simulink model "Improved_EKFSim"  (R2023b)
settings: Solver=VariableStepAuto  StartTime=0.0  StopTime=6000  RelTol=1e-3
libraries: commchan3 x2, SignalEditorBlockLib x1
settings Model: Creator=Lenovo  LastModifiedBy=dell
settings SolverCC: AlgebraicLoopSolver=TrustRegion
settings DataIOCC: ReturnWorkspaceOutputs=off
settings DebuggingCC: UnconnectedInputMsg=warning  UnconnectedOutputMsg=warning  UnconnectedLineMsg=warning  ArithmeticOperatorsInVariantConditions=warning
settings ModelReferenceCC: EnableRefExpFcnMdlSchedulingChecks=on
settings SFSimCC: SimUseLocalCustomCode=off  CustomCodeUndefinedFunction=UseInterfaceOnly
settings RTWCC: RTWUseLocalCustomCode=off  DLArmComputeVersion=19.05

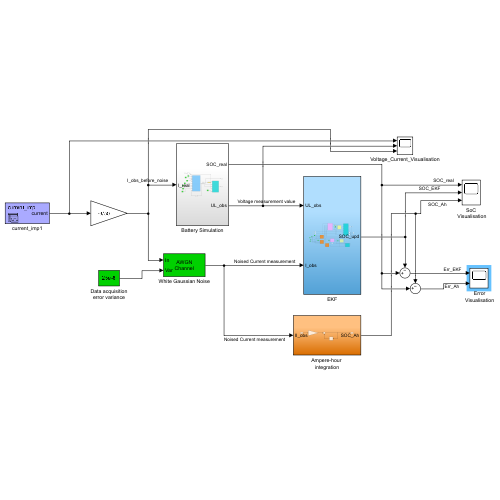
[thumbnail: Simulink's stored preview of the top-level diagram]
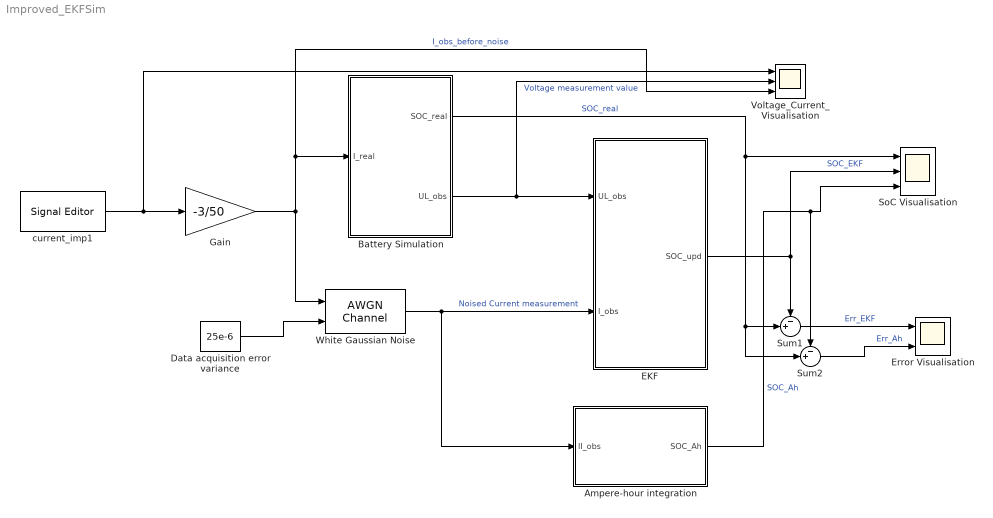
== system Improved_EKFSim ==
  "  Error Visualisation" : Scope  NumInputPorts=2
  " SoC Visualisation" : Scope  NumInputPorts=3
  Ampere-hour integration : Subsystem
  Battery Simulation : Subsystem
  Data acquisition error variance : Constant  Value=25e-6
  EKF : Subsystem
  Gain : Gain  Gain=-3/50
  Sum1 : Sum  Inputs=-+|
  Sum2 : Sum  Inputs=-+|
  Voltage_Current_Visualisation : Scope  NumInputPorts=3
  White Gaussian Noise : commchan3/AWGN Channel  LegacyMode=on  NoiseMethod="Signal to noise ratio  (SNR)"  noiseMode=Variance from port  EbNo=10  EsNo=10  SNR=10  BitsPerSymbol=1  SignalPower=1  SamplesPerSymbol=1  SymbolPeriod=1  VarianceSource=Parameter  Variance=1  RandomStream=Global stream  Seed=1  SimulateUsing=Code generation
  current_imp1 : SignalEditorBlockLib/Signal Editor  FileName=C:\Users\dell\Downloads\BMS_EKF\scripts\dataset.mat  ActiveScenario=current_imp  ActiveSignal=current  IsBus=off  OutputBusObjectStr=Bus: BusObject  SampleTime=0  OutputAfterFinalValue=Extrapolation  Unit=inherit  PreserveSignalName=on  ApplySigPropsToAllScenarios=on  ApplySigPropsToAllSignals=off
  wires:
  White Gaussian Noise/1 -> EKF/2(I_obs), Ampere-hour integration/1(II_obs)  "Noised Current measurement"
  EKF/1(SOC_upd) -> Sum1/1, " SoC Visualisation"/2  "SOC_EKF"
  Battery Simulation/2(UL_obs) -> Voltage_Current_Visualisation/2, EKF/1(UL_obs)  "Voltage measurement value"
  Battery Simulation/1(SOC_real) -> Sum2/2, Sum1/2, " SoC Visualisation"/1  "SOC_real"
  Gain/1 -> Voltage_Current_Visualisation/3, Battery Simulation/1(I_real), White Gaussian Noise/1  "I_obs_before_noise"
  Ampere-hour integration/1(SOC_Ah) -> " SoC Visualisation"/3, Sum2/1  "SOC_Ah"
  Sum1/1 -> "  Error Visualisation"/1  "Err_EKF"
  Sum2/1 -> "  Error Visualisation"/2  "Err_Ah"
  Data acquisition error variance/1 -> White Gaussian Noise/2
  current_imp1/1 -> Voltage_Current_Visualisation/1, Gain/1

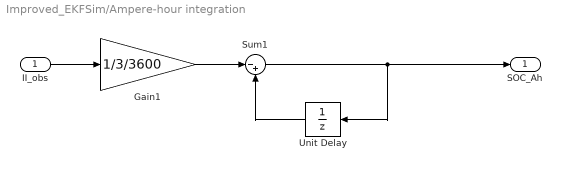
== system Improved_EKFSim/Ampere-hour integration ==
  II_obs : Inport
  Gain1 : Gain  Gain=1/3/3600
  Sum1 : Sum  Inputs=|-+
  Unit Delay : UnitDelay  InitialCondition=1  HasFrameUpgradeWarning=on
  SOC_Ah : Outport  VectorParamsAs1DForOutWhenUnconnected=off
  wires:
  Gain1/1 -> Sum1/1
  Sum1/1 -> SOC_Ah/1, Unit Delay/1
  II_obs/1 -> Gain1/1
  Unit Delay/1 -> Sum1/2

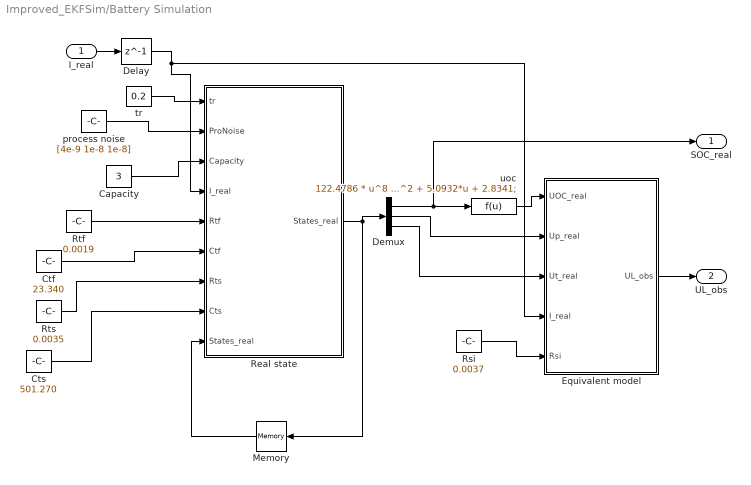
== system Improved_EKFSim/Battery Simulation ==
  I_real : Inport
  Capacity : Constant  Value=3
  Ctf : Constant  Value=23.340
  Cts : Constant  Value=501.270
  Delay : Delay  DelayLength=1  InitialCondition=0  SampleTime=0.1
  Demux : Demux  Outputs=3
  Equivalent model : Subsystem  TreatAsAtomicUnit=on
  Memory : Memory  InitialCondition=[1;0;0]
  Real state : MATLAB Function  TreatAsAtomicUnit=on
  Rsi : Constant  Value=0.0037
  Rtf : Constant  Value=0.0019
  Rts : Constant  Value=0.0035
  process noise : Constant  Value=[4e-9 1e-8 1e-8]
  tr : Constant  Value=0.2
  uoc : Fcn  Expr=122.4786 * u^8 - 401.4734 * u^7 + 485.6818 * u^6 -239.2806 * u^5 + 3.7304 * u^4 + 44.9020 * u^3 - 19.8057 * u^2 + 5.0932*u + 2.8341;
  SOC_real : Outport  VectorParamsAs1DForOutWhenUnconnected=off
  UL_obs : Outport  Port=2  VectorParamsAs1DForOutWhenUnconnected=off
  wires:
  Demux/2 -> Equivalent model/2(Up_real)
  Rtf/1 -> Real state/5(Rtf)
  tr/1 -> Real state/1(tr)
  Real state/1(States_real) -> Demux/1, Memory/1
  Rsi/1 -> Equivalent model/5(Rsi)
  Ctf/1 -> Real state/6(Ctf)
  Capacity/1 -> Real state/3(Capacity)
  uoc/1 -> Equivalent model/1(UOC_real)
  Memory/1 -> Real state/9("States_real ")
  process noise/1 -> Real state/2(ProNoise)
  Equivalent model/1(UL_obs) -> UL_obs/1
  Delay/1 -> Real state/4(I_real), Equivalent model/4(I_real)
  Demux/1 -> uoc/1, SOC_real/1
  I_real/1 -> Delay/1
  Rts/1 -> Real state/7(Rts)
  Cts/1 -> Real state/8(Cts)
  Demux/3 -> Equivalent model/3(Ut_real)

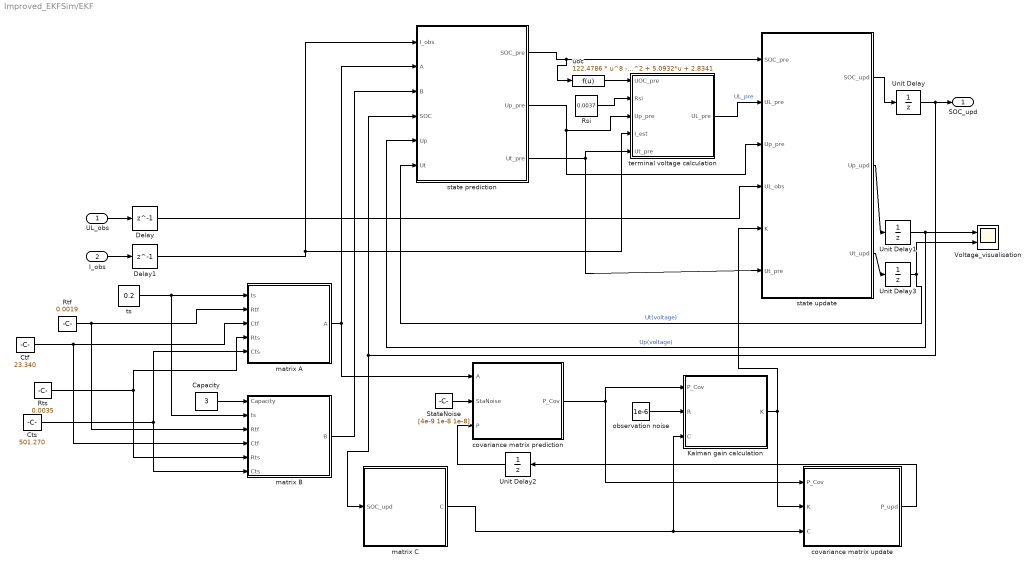
== system Improved_EKFSim/EKF ==
  UL_obs : Inport
  I_obs : Inport  Port=2
  Capacity : Constant  Value=3
  Ctf : Constant  Value=23.340
  Cts : Constant  Value=501.270
  Delay : Delay  DelayLength=1  InitialCondition=0  SampleTime=1
  Delay1 : Delay  DelayLength=1  InitialCondition=0  SampleTime=1
  Kalman gain calculation : MATLAB Function  TreatAsAtomicUnit=on
  Rsi : Constant  Value=0.0037
  Rtf : Constant  Value=0.0019
  Rts : Constant  Value=0.0035
  StateNoise : Constant  Value=[4e-9 1e-8 1e-8]
  Unit Delay : UnitDelay  InitialCondition=1  HasFrameUpgradeWarning=on
  Unit Delay1 : UnitDelay  HasFrameUpgradeWarning=on
  Unit Delay2 : UnitDelay  InitialCondition=[0 0 0;0 0 0; 0 0 0]  HasFrameUpgradeWarning=on
  Unit Delay3 : UnitDelay  HasFrameUpgradeWarning=on
  Voltage_visualisation : Scope  NumInputPorts=2
  covariance matrix prediction : MATLAB Function  TreatAsAtomicUnit=on
  covariance matrix update : MATLAB Function  TreatAsAtomicUnit=on
  matrix A : Subsystem  TreatAsAtomicUnit=on
  matrix B : Subsystem  TreatAsAtomicUnit=on
  matrix C : Subsystem  TreatAsAtomicUnit=on
  observation noise : Constant  Value=1e-6
  state prediction : Subsystem
  state update : Subsystem
  terminal voltage calculation : Subsystem  TreatAsAtomicUnit=on
  ts : Constant  Value=0.2
  uoc : Fcn  Expr=122.4786 * u^8 - 401.4734 * u^7 + 485.6818 * u^6 -239.2806 * u^5 + 3.7304 * u^4 + 44.9020 * u^3 - 19.8057 * u^2 + 5.0932*u + 2.8341
  SOC_upd : Outport  VectorParamsAs1DForOutWhenUnconnected=off
  wires:
  matrix C/1(" C") -> covariance matrix update/3(C), Kalman gain calculation/3(C)
  matrix A/1(A) -> state prediction/2(A), covariance matrix prediction/1(A)
  StateNoise/1 -> covariance matrix prediction/2(StaNoise)
  Kalman gain calculation/1(K) -> covariance matrix update/2(K), state update/5(K)
  ts/1 -> matrix B/2(ts), matrix A/1(ts)
  covariance matrix update/1(P_upd) -> Unit Delay2/1
  Capacity/1 -> matrix B/1(Capacity)
  I_obs/1 -> Delay1/1
  observation noise/1 -> Kalman gain calculation/2(R)
  UL_obs/1 -> Delay/1
  uoc/1 -> terminal voltage calculation/1(UOC_pre)
  Delay1/1 -> state prediction/1(I_obs), terminal voltage calculation/4(I_est)
  state update/2(Up_upd) -> Unit Delay1/1
  state update/1(SOC_upd) -> Unit Delay/1
  terminal voltage calculation/1(UL_pre) -> state update/2(UL_pre)  "UL_pre"
  Delay/1 -> state update/4(UL_obs)
  state prediction/1(SOC_pre) -> uoc/1, state update/1(SOC_pre)
  state prediction/2(Up_pre) -> state update/3(Up_pre), terminal voltage calculation/3(Up_pre)
  Unit Delay/1 -> state prediction/4(SOC), matrix C/1(SOC_upd), SOC_upd/1
  Unit Delay1/1 -> state prediction/5(Up), Voltage_visualisation/1  "Up(voltage)"
  matrix B/1(B) -> state prediction/3(B)
  covariance matrix prediction/1(P_Cov) -> covariance matrix update/1(P_Cov), Kalman gain calculation/1(P_Cov)
  Unit Delay2/1 -> covariance matrix prediction/3(P)
  Rtf/1 -> matrix B/3(Rtf), matrix A/2(Rtf)
  Ctf/1 -> matrix B/4(Ctf), matrix A/3(Ctf)
  Rts/1 -> matrix A/4(Rts), matrix B/5(Rts)
  Cts/1 -> matrix B/6(Cts), matrix A/5(Cts)
  Rsi/1 -> terminal voltage calculation/2(Rsi)
  state prediction/3(Ut_pre) -> state update/6(Ut_pre), terminal voltage calculation/5(Ut_pre)
  state update/3(Ut_upd) -> Unit Delay3/1
  Unit Delay3/1 -> Voltage_visualisation/2, state prediction/6(Ut)  "Ut(voltage)"

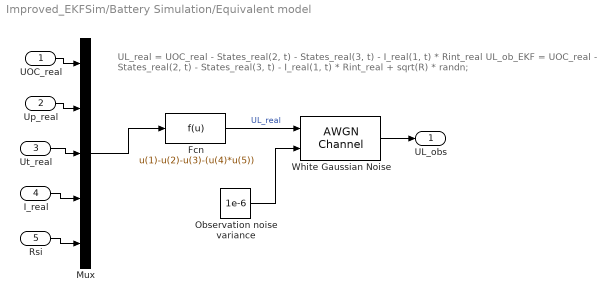
== system Improved_EKFSim/Battery Simulation/Equivalent model ==
  note: UL_real = UOC_real - States_real(2, t) - States_real(3, t) - I_real(1, t) * Rint_real
      | UL_ob_EKF = UOC_real - States_real(2, t) - States_real(3, t) - I_real(1, t) * Rint_real + sqrt(R) * randn;
  UOC_real : Inport
  Up_real : Inport  Port=2
  Ut_real : Inport  Port=3
  I_real : Inport  Port=4
  Rsi : Inport  Port=5
  Fcn : Fcn  Expr=u(1)-u(2)-u(3)-(u(4)*u(5))
  Mux : Mux  Inputs=5
  Observation noise variance : Constant  Value=1e-6
  White Gaussian Noise : commchan3/AWGN Channel  LegacyMode=on  NoiseMethod="Signal to noise ratio  (SNR)"  noiseMode=Variance from port  EbNo=10  EsNo=10  SNR=10  BitsPerSymbol=1  SignalPower=1  SamplesPerSymbol=1  SymbolPeriod=1  VarianceSource=Parameter  Variance=1  RandomStream=Global stream  Seed=1  SimulateUsing=Code generation
  UL_obs : Outport  VectorParamsAs1DForOutWhenUnconnected=off
  wires:
  Fcn/1 -> White Gaussian Noise/1  "UL_real"
  Mux/1 -> Fcn/1
  UOC_real/1 -> Mux/1
  Up_real/1 -> Mux/2
  I_real/1 -> Mux/4
  Rsi/1 -> Mux/5
  White Gaussian Noise/1 -> UL_obs/1
  Observation noise variance/1 -> White Gaussian Noise/2
  Ut_real/1 -> Mux/3

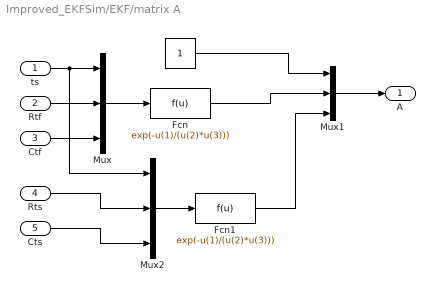
== system Improved_EKFSim/EKF/matrix A ==
  ts : Inport
  Rtf : Inport  Port=2
  Ctf : Inport  Port=3
  Rts : Inport  Port=4
  Cts : Inport  Port=5
  " " : Constant
  Fcn : Fcn  Expr=exp(-u(1)/(u(2)*u(3)))
  Fcn1 : Fcn  Expr=exp(-u(1)/(u(2)*u(3)))
  Mux : Mux  Inputs=3
  Mux1 : Mux  Inputs=3
  Mux2 : Mux  Inputs=3
  A : Outport  VectorParamsAs1DForOutWhenUnconnected=off
  wires:
  Rtf/1 -> Mux/2
  Fcn/1 -> Mux1/2
  ts/1 -> Mux2/1, Mux/1
  Ctf/1 -> Mux/3
  Mux/1 -> Fcn/1
  " "/1 -> Mux1/1
  Mux1/1 -> A/1
  Rts/1 -> Mux2/2
  Cts/1 -> Mux2/3
  Fcn1/1 -> Mux1/3
  Mux2/1 -> Fcn1/1

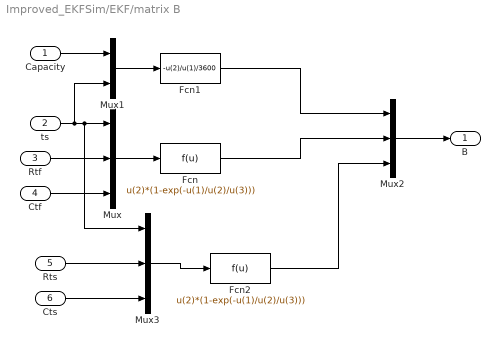
== system Improved_EKFSim/EKF/matrix B ==
  Capacity : Inport
  ts : Inport  Port=2
  Rtf : Inport  Port=3
  Ctf : Inport  Port=4
  Rts : Inport  Port=5
  Cts : Inport  Port=6
  Fcn : Fcn  Expr=u(2)*(1-exp(-u(1)/u(2)/u(3)))
  Fcn1 : Fcn  Expr=-u(2)/u(1)/3600
  Fcn2 : Fcn  Expr=u(2)*(1-exp(-u(1)/u(2)/u(3)))
  Mux : Mux  Inputs=3
  Mux1 : Mux  Inputs=2
  Mux2 : Mux  Inputs=3
  Mux3 : Mux  Inputs=3
  B : Outport  VectorParamsAs1DForOutWhenUnconnected=off
  wires:
  Rtf/1 -> Mux/2
  ts/1 -> Mux1/2, Mux3/1, Mux/1
  Ctf/1 -> Mux/3
  Mux/1 -> Fcn/1
  Capacity/1 -> Mux1/1
  Mux1/1 -> Fcn1/1
  Fcn/1 -> Mux2/2
  Fcn1/1 -> Mux2/1
  Mux2/1 -> B/1
  Rts/1 -> Mux3/2
  Cts/1 -> Mux3/3
  Fcn2/1 -> Mux2/3
  Mux3/1 -> Fcn2/1

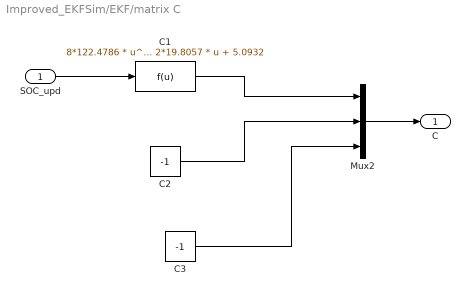
== system Improved_EKFSim/EKF/matrix C ==
  SOC_upd : Inport
  C1 : Fcn  Expr=8*122.4786 * u^7 - 7*401.4734 * u^6 + 6*485.6818 * u^5 -5*239.2806 * u^4 + 4*3.7304 * u^3 + 3*44.9020 * u^2 - 2*19.8057 * u + 5.0932
  C2 : Constant  Value=-1
  C3 : Constant  Value=-1
  Mux2 : Mux  Inputs=3
  " C" : Outport  VectorParamsAs1DForOutWhenUnconnected=off
  wires:
  C1/1 -> Mux2/1
  C2/1 -> Mux2/2
  Mux2/1 -> " C"/1
  SOC_upd/1 -> C1/1
  C3/1 -> Mux2/3

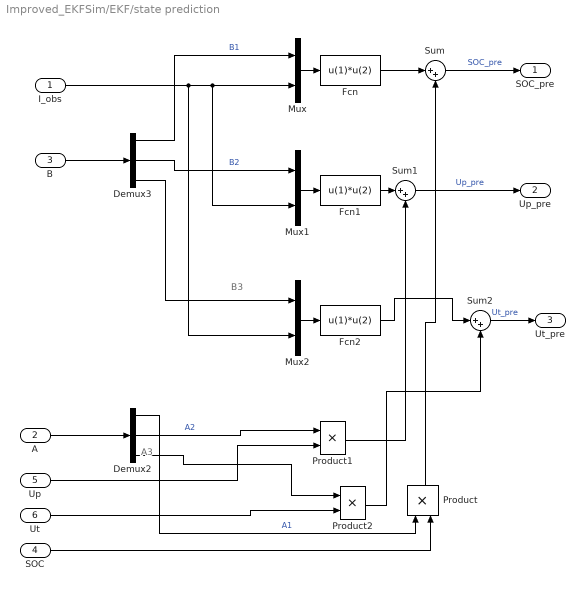
== system Improved_EKFSim/EKF/state prediction ==
  note: B3
  note: A3
  I_obs : Inport
  A : Inport  Port=2
  B : Inport  Port=3
  SOC : Inport  Port=4
  Up : Inport  Port=5
  Ut : Inport  Port=6
  Demux2 : Demux  Outputs=3
  Demux3 : Demux  Outputs=3
  Fcn : Fcn  Expr=u(1)*u(2)
  Fcn1 : Fcn  Expr=u(1)*u(2)
  Fcn2 : Fcn  Expr=u(1)*u(2)
  Mux : Mux  Inputs=2
  Mux1 : Mux  Inputs=2
  Mux2 : Mux  Inputs=2
  Product : Product
  Product1 : Product
  Product2 : Product
  Sum : Sum  Inputs=|++
  Sum1 : Sum  Inputs=|++
  Sum2 : Sum  Inputs=|++
  SOC_pre : Outport  VectorParamsAs1DForOutWhenUnconnected=off
  Up_pre : Outport  Port=2  VectorParamsAs1DForOutWhenUnconnected=off
  Ut_pre : Outport  Port=3  VectorParamsAs1DForOutWhenUnconnected=off
  wires:
  Fcn/1 -> Sum/1
  Demux2/2 -> Product1/1  "A2"
  A/1 -> Demux2/1
  Demux3/1 -> Mux/1  "B1"
  Demux2/1 -> Product/1  "A1"
  SOC/1 -> Product/2
  Fcn1/1 -> Sum1/1
  Mux/1 -> Fcn/1
  Mux1/1 -> Fcn1/1
  Product/1 -> Sum/2
  Demux3/2 -> Mux1/1  "B2"
  Sum1/1 -> Up_pre/1  "Up_pre"
  I_obs/1 -> Mux2/2, Mux1/2, Mux/2
  Up/1 -> Product1/2
  Product1/1 -> Sum1/2
  Sum/1 -> SOC_pre/1  "SOC_pre"
  B/1 -> Demux3/1
  Demux3/3 -> Mux2/1
  Mux2/1 -> Fcn2/1
  Sum2/1 -> Ut_pre/1  "Ut_pre"
  Fcn2/1 -> Sum2/1
  Demux2/3 -> Product2/1
  Ut/1 -> Product2/2
  Product2/1 -> Sum2/2

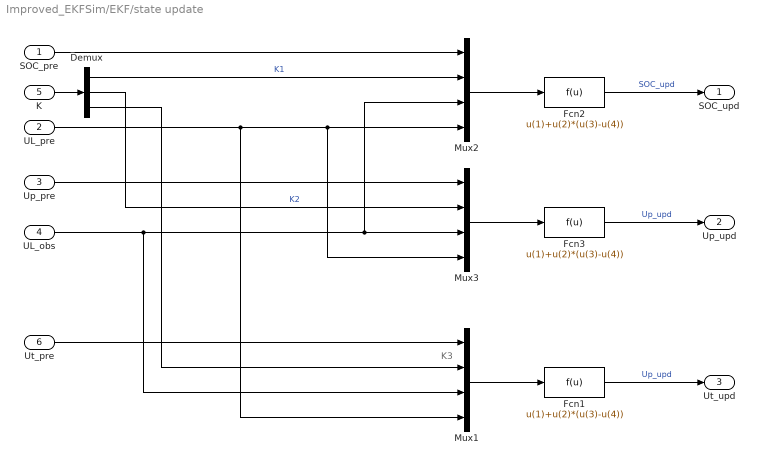
== system Improved_EKFSim/EKF/state update ==
  note: K3
  SOC_pre : Inport
  UL_pre : Inport  Port=2
  Up_pre : Inport  Port=3
  UL_obs : Inport  Port=4
  K : Inport  Port=5
  Ut_pre : Inport  Port=6
  Demux : Demux  Outputs=3
  Fcn1 : Fcn  Expr=u(1)+u(2)*(u(3)-u(4))
  Fcn2 : Fcn  Expr=u(1)+u(2)*(u(3)-u(4))
  Fcn3 : Fcn  Expr=u(1)+u(2)*(u(3)-u(4))
  Mux1 : Mux
  Mux2 : Mux
  Mux3 : Mux
  SOC_upd : Outport  VectorParamsAs1DForOutWhenUnconnected=off
  Up_upd : Outport  Port=2  VectorParamsAs1DForOutWhenUnconnected=off
  Ut_upd : Outport  Port=3  VectorParamsAs1DForOutWhenUnconnected=off
  wires:
  Fcn3/1 -> Up_upd/1  "Up_upd"
  Demux/1 -> Mux2/2  "K1"
  Demux/2 -> Mux3/2  "K2"
  Mux2/1 -> Fcn2/1
  Mux3/1 -> Fcn3/1
  K/1 -> Demux/1
  UL_obs/1 -> Mux1/3, Mux3/3, Mux2/3
  Up_pre/1 -> Mux3/1
  SOC_pre/1 -> Mux2/1
  Fcn2/1 -> SOC_upd/1  "SOC_upd"
  Ut_pre/1 -> Mux1/1
  Mux1/1 -> Fcn1/1
  Fcn1/1 -> Ut_upd/1  "Up_upd"
  Demux/3 -> Mux1/2
  UL_pre/1 -> Mux1/4, Mux3/4, Mux2/4

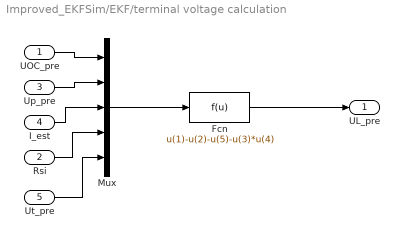
== system Improved_EKFSim/EKF/terminal voltage calculation ==
  UOC_pre : Inport
  Rsi : Inport  Port=2
  Up_pre : Inport  Port=3
  I_est : Inport  Port=4
  Ut_pre : Inport  Port=5
  Fcn : Fcn  Expr=u(1)-u(2)-u(5)-u(3)*u(4)
  Mux : Mux  Inputs=5
  UL_pre : Outport  VectorParamsAs1DForOutWhenUnconnected=off
  wires:
  I_est/1 -> Mux/3
  Up_pre/1 -> Mux/2
  Rsi/1 -> Mux/4
  Mux/1 -> Fcn/1
  Fcn/1 -> UL_pre/1
  UOC_pre/1 -> Mux/1
  Ut_pre/1 -> Mux/5

== matlab function Improved_EKFSim/Battery Simulation/Real state ==
  data: tr input; States_real output; ProNoise input; Capacity input; I_real input; Rtf input; Ctf input; Rts input; Cts input; States_real input
function States_real = StatReal(tr, ProNoise, Capacity, I_real, Rtf, Ctf,Rts, Cts, States_real)
%     tao = Rp1 * Cp1;
    Qs = ProNoise(1);
    Qu = ProNoise(2);
    Qt = ProNoise(3);
    A1=1;
    tao1 = Rtf * Ctf;
    A2 = exp(-tr / tao1);
    tao2 = Rts * Cts;
    A3 = exp(-tr / tao2);

    A =[A1 0 0; 0 A2 0; 0 0 A3];  % State transformation matrix

    B1 = - tr / (Capacity * 3600);
    B2 = Rtf * (1 - exp(-tr / tao1));
    B3 = Rts * (1 - exp(-tr / tao2));
    B = [B1; B2; B3];  % Input control matrix
    States_real = A*States_real + B*I_real + [sqrt(Qs)*randn ;sqrt(Qu)*randn ;sqrt(Qt)*randn];  % The actual process simulation updates every 0.1 seconds.

== matlab function Improved_EKFSim/EKF/covariance matrix prediction ==
  data: A input; P_Cov output; StaNoise input; P input
function P_Cov = CovMat(A, StaNoise, P)
A1 = [A(1) 0 0;0 A(2) 0; 0 0 A(3)];
Qs = StaNoise(1);
Qu = StaNoise(2);
Qt = StaNoise(3);

P1 = [P(1) P(2) P(3); P(4) P(5) P(6); P(7) P(8) P(9)];
P2 = A1*P1*A1' + [Qs 0 0;0 Qu 0; 0 0 Qt];  % covariance matrix prediction
P_Cov = [P2(1,1) P2(1,2) P2(1,3); P2(2,1) P2(2,2) P2(2,3); P2(3,1) P2(3,2) P2(3,3)];

== matlab function Improved_EKFSim/EKF/Kalman gain calculation ==
  data: P_Cov input; R input; C input; K output
function K = KalmanGain(P_Cov, R, C)
C1 = [C(1) C(2) C(3)];
P = [P_Cov(1) P_Cov(2) P_Cov(3); P_Cov(4) P_Cov(5) P_Cov(6); P_Cov(7) P_Cov(8) P_Cov(9)];
K = P*C1'* (C1*P*C1'+R)^(-1);  % Gain

== matlab function Improved_EKFSim/EKF/covariance matrix update ==
  data: P_Cov input; K input; C input; P_upd output
function P_upd = CovUpd(P_Cov, K, C)
C = [C(1) C(2) C(3)];
P = [P_Cov(1) P_Cov(2) P_Cov(3); P_Cov(4) P_Cov(5) P_Cov(6); P_Cov(7) P_Cov(8) P_Cov(9)];
P1 = P - K * C * P;  % Covariance matrix update
P_upd = [P1(1,1) P1(1,2) P1(1,3); P1(2,1) P1(2,2) P1(2,3); P1(3,1) P1(3,2) P1(3,3)];
